simulink model "robotaz00"  (R2017a)
settings: Solver=VariableStepAuto  StartTime=0.0  StopTime=10.0  RelTol=1e-3
undefined symbols (not defined in the file or in its folder): Antebrazo, BASE, BrazoCOPIA, Codo, Hombrocopia, mesa, robotaz, RootGround, RootPart
libraries: mblibv1 x41
settings Model: Creator=ckarl  LastModifiedBy=ckarl
settings SimMechanicsCC: VisOnUpdateDiagram=on  VisDuringSimulation=on

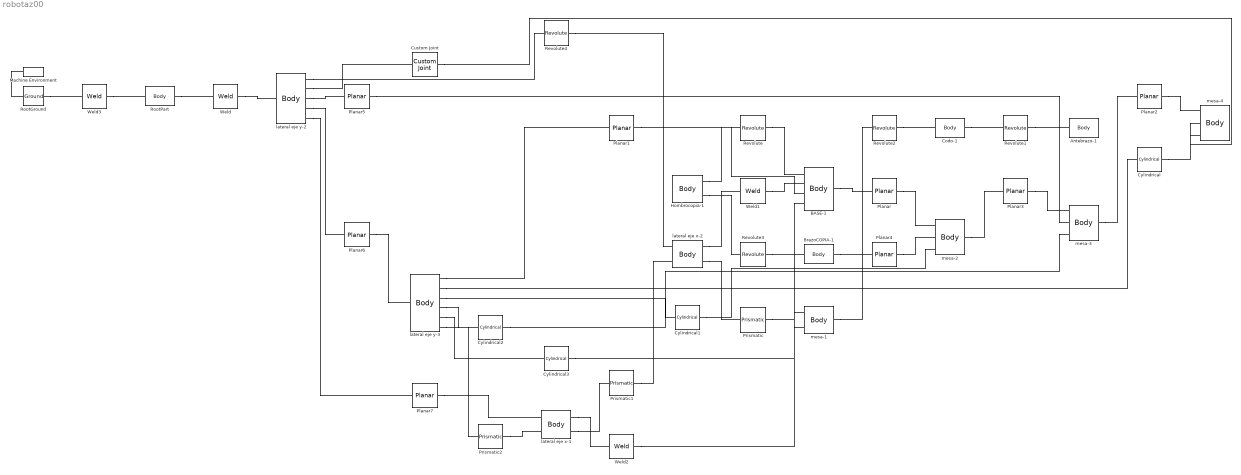
== system robotaz00 ==
  Antebrazo-1 : mblibv1/Bodies/Body  LConnTagsString=CS2  UpdateFromCAD=on  PMImportedID=Antebrazo-1  DialogClass=MechanicalBodyBlock  Mass=6.4203  MassUnits=kg  InertiaUnits=kg*m^2  Inertia=[0.103996,-2.98129e-06,0.00137963;-2.98129e-06,0.0987801,7.6206e-06;0.00137963,7.6206e-06,0.0190701]  Shape=Cylinder  ShapeDims=[1 1]  ShapeUnits=m  ShapeUse=false  Density=1  DensityUnits=kg/m^3  DensityUse=false  GraphicsMode=GFXFILE  GraphicsFileName=robotaz - Antebrazo-1.STL  BodyColorSelMode=COLORPALETTE  BodyColor=[0.792157;0.819608;0.933333]  AttachedToCS=CS1  CG=Right$CG$[-0.0536428 0.244253 1.19012]$WORLD$WORLD$m$[-0.573445 -0.772871 -0.271718;0.0436025 0.302406 -0.952181;0.818083 -0.557871 -0.139714]$3x3 Transform$rad$WORLD$false$Antebrazo-1::CG(AUTOGEN)  WorkingFrames=Right$CS1$[0.0431037 0.587411 1.24209]$WORLD$WORLD$m$[-0.573445 -0.772871 -0.271718;0.0436025 0.302406 -0.952181;0.818083 -0.557871 -0.139714]$3x3 Transform$rad$WORLD$false$Antebrazo-1::CS1(AUTOGEN)#Left$CS2$[0.000440757 0.437907 1.22016]$WORLD$WORLD$m$[1 0 0;0 1 0;0 0 1]$3x3 Transform$rad$WORLD$true$Antebrazo-1:-:Codo-1::Antebrazo-1(AUTOGEN)  CGPos=[-0.0536428 0.244253 1.19012]  CGRot=[-0.573445 -0.772871 -0.271718;0.0436025 0.302406 -0.952181;0.818083 -0.557871 -0.139714]  CS0Pos=[]  CS0Rot=[]  CS1Pos=[0.0431037 0.587411 1.24209]  CS1Rot=[-0.573445 -0.772871 -0.271718;0.0436025 0.302406 -0.952181;0.818083 -0.557871 -0.139714]  CS2Pos=[0.000440757 0.437907 1.22016]  CS2Rot=[1 0 0;0 1 0;0 0 1]  CS3Pos=[]  CS3Rot=[]  CS4Pos=[]  CS4Rot=[]  CS5Pos=[]  CS5Rot=[]  CS6Pos=[]  CS6Rot=[]  CS7Pos=[]  CS7Rot=[]  CS8Pos=[]  CS8Rot=[]  CS9Pos=[]  CS9Rot=[]  CS10Pos=[]  CS10Rot=[]  CS11Pos=[]  CS11Rot=[]  CS12Pos=[]  CS12Rot=[]  CS13Pos=[]  CS13Rot=[]  CS14Pos=[]  CS14Rot=[]  CS15Pos=[]  CS15Rot=[]  CS16Pos=[]  CS16Rot=[]  CS17Pos=[]  CS17Rot=[]  CS18Pos=[]  CS18Rot=[]  CS19Pos=[]  CS19Rot=[]  CS20Pos=[]  CS20Rot=[]
      settings: SourceProductName=Simscape Multibody  SourceProductBaseCode=MS
  BASE-1 : mblibv1/Bodies/Body  LConnTagsString=CS2|CS3|CS5|CS6  RConnTagsString=CS4  UpdateFromCAD=on  PMImportedID=BASE-1  DialogClass=MechanicalBodyBlock  Mass=23.2061  MassUnits=kg  InertiaUnits=kg*m^2  Inertia=[0.362789,0.0180466,-0.00054238;0.0180466,0.257111,-0.000428667;-0.00054238,-0.000428667,0.35504]  Shape=Cylinder  ShapeDims=[1 1]  ShapeUnits=m  ShapeUse=false  Density=1  DensityUnits=kg/m^3  DensityUse=false  GraphicsMode=GFXFILE  GraphicsFileName=robotaz - BASE-1.STL  BodyColorSelMode=COLORPALETTE  BodyColor=[1;0.54902;0]  AttachedToCS=CS1  CG=Right$CG$[0.148607 0.398211 0.794801]$WORLD$WORLD$m$[1 0 0;0 1 0;0 0 1]$3x3 Transform$rad$WORLD$false$BASE-1::CG(AUTOGEN)  WorkingFrames=Right$CS1$[0.140125 0.230213 0.795]$WORLD$WORLD$m$[1 0 0;0 1 0;0 0 1]$3x3 Transform$rad$WORLD$false$BASE-1::CS1(AUTOGEN)#Left$CS2$[0.140125 0.580213 0.795]$WORLD$WORLD$m$[1 0 0;0 1 0;0 0 1]$3x3 Transform$rad$WORLD$true$BASE-1:-:Hombrocopia-1::BASE-1(AUTOGEN)#Left$CS3$[-0.0148746 0.0738361 0.795]$WORLD$WORLD$m$[1 0 0;0 1 0;0 0 1]$3x3 Transform$rad$WORLD$true$BASE-1:-:lateral eje x-2::BASE-1(AUTOGEN)#Right$CS4$[0.140125 0.230213 0.795]$WORLD$WORLD$m$[1 0 0;0 1 0;0 0 1]$3x3 Transform$rad$WORLD$true$BASE-1:-:mesa-2::BASE-1(AUTOGEN)#Left$CS5$[0.310125 -0.0917867 0.945]$WORLD$WORLD$m$[1 0 0;0 1 0;0 0 1]$3x3 Transform$rad$WORLD$true$BASE-1:-:lateral eje y-3::BASE-1(AUTOGEN)#Left$CS6$[0.295125 0.0738361 0.795]$WORLD$WORLD$m$[1 0 0;0 1 0;0 0 1]$3x3 Transform$rad$WORLD$true$BASE-1:-:lateral eje x-1::BASE-1(AUTOGEN)  CGPos=[0.148607 0.398211 0.794801]  CGRot=[1 0 0;0 1 0;0 0 1]  CS0Pos=[]  CS0Rot=[]  CS1Pos=[0.140125 0.230213 0.795]  CS1Rot=[1 0 0;0 1 0;0 0 1]  CS2Pos=[0.140125 0.580213 0.795]  CS2Rot=[1 0 0;0 1 0;0 0 1]  CS3Pos=[-0.0148746 0.0738361 0.795]  CS3Rot=[1 0 0;0 1 0;0 0 1]  CS4Pos=[0.140125 0.230213 0.795]  CS4Rot=[1 0 0;0 1 0;0 0 1]  CS5Pos=[0.310125 -0.0917867 0.945]  CS5Rot=[1 0 0;0 1 0;0 0 1]  CS6Pos=[0.295125 0.0738361 0.795]  CS6Rot=[1 0 0;0 1 0;0 0 1]  CS7Pos=[]  CS7Rot=[]  CS8Pos=[]  CS8Rot=[]  CS9Pos=[]  CS9Rot=[]  CS10Pos=[]  CS10Rot=[]  CS11Pos=[]  CS11Rot=[]  CS12Pos=[]  CS12Rot=[]  CS13Pos=[]  CS13Rot=[]  CS14Pos=[]  CS14Rot=[]  CS15Pos=[]  CS15Rot=[]  CS16Pos=[]  CS16Rot=[]  CS17Pos=[]  CS17Rot=[]  CS18Pos=[]  CS18Rot=[]  CS19Pos=[]  CS19Rot=[]  CS20Pos=[]  CS20Rot=[]
      settings: SourceProductName=Simscape Multibody  SourceProductBaseCode=MS
  BrazoCOPIA-1 : mblibv1/Bodies/Body  LConnTagsString=CS3  RConnTagsString=CS2  UpdateFromCAD=on  PMImportedID=BrazoCOPIA-1  DialogClass=MechanicalBodyBlock  Mass=31.6067  MassUnits=kg  InertiaUnits=kg*m^2  Inertia=[3.43366,-7.27901e-06,-0.0175763;-7.27901e-06,3.34876,-4.89263e-05;-0.0175763,-4.89263e-05,0.211578]  Shape=Cylinder  ShapeDims=[1 1]  ShapeUnits=m  ShapeUse=false  Density=1  DensityUnits=kg/m^3  DensityUse=false  GraphicsMode=GFXFILE  GraphicsFileName=robotaz - BrazoCOPIA-1.STL  BodyColorSelMode=COLORPALETTE  BodyColor=[0.792157;0.819608;0.933333]  AttachedToCS=CS1  CG=Right$CG$[-0.109909 1.05734 1.38561]$WORLD$WORLD$m$[0.45728 -0.87962 -0.131012;0 -0.147317 0.989089;-0.889323 -0.45229 -0.067365]$3x3 Transform$rad$WORLD$false$BrazoCOPIA-1::CG(AUTOGEN)  WorkingFrames=Right$CS1$[-0.15801 1.37772 1.37482]$WORLD$WORLD$m$[0.45728 -0.87962 -0.131012;0 -0.147317 0.989089;-0.889323 -0.45229 -0.067365]$3x3 Transform$rad$WORLD$false$BrazoCOPIA-1::CS1(AUTOGEN)#Right$CS2$[-0.0120448 0.586448 1.34867]$WORLD$WORLD$m$[1 0 0;0 1 0;0 0 1]$3x3 Transform$rad$WORLD$true$BrazoCOPIA-1:-:Codo-1::BrazoCOPIA-1(AUTOGEN)#Left$CS3$[-0.116855 1.37772 1.29478]$WORLD$WORLD$m$[1 0 0;0 1 0;0 0 1]$3x3 Transform$rad$WORLD$true$BrazoCOPIA-1:-:Hombrocopia-1::BrazoCOPIA-1(AUTOGEN)  CGPos=[-0.109909 1.05734 1.38561]  CGRot=[0.45728 -0.87962 -0.131012;0 -0.147317 0.989089;-0.889323 -0.45229 -0.067365]  CS0Pos=[]  CS0Rot=[]  CS1Pos=[-0.15801 1.37772 1.37482]  CS1Rot=[0.45728 -0.87962 -0.131012;0 -0.147317 0.989089;-0.889323 -0.45229 -0.067365]  CS2Pos=[-0.0120448 0.586448 1.34867]  CS2Rot=[1 0 0;0 1 0;0 0 1]  CS3Pos=[-0.116855 1.37772 1.29478]  CS3Rot=[1 0 0;0 1 0;0 0 1]  CS4Pos=[]  CS4Rot=[]  CS5Pos=[]  CS5Rot=[]  CS6Pos=[]  CS6Rot=[]  CS7Pos=[]  CS7Rot=[]  CS8Pos=[]  CS8Rot=[]  CS9Pos=[]  CS9Rot=[]  CS10Pos=[]  CS10Rot=[]  CS11Pos=[]  CS11Rot=[]  CS12Pos=[]  CS12Rot=[]  CS13Pos=[]  CS13Rot=[]  CS14Pos=[]  CS14Rot=[]  CS15Pos=[]  CS15Rot=[]  CS16Pos=[]  CS16Rot=[]  CS17Pos=[]  CS17Rot=[]  CS18Pos=[]  CS18Rot=[]  CS19Pos=[]  CS19Rot=[]  CS20Pos=[]  CS20Rot=[]
      settings: SourceProductName=Simscape Multibody  SourceProductBaseCode=MS
  Codo-1 : mblibv1/Bodies/Body  LConnTagsString=CS3  RConnTagsString=CS2  UpdateFromCAD=on  PMImportedID=Codo-1  DialogClass=MechanicalBodyBlock  Mass=7.50271  MassUnits=kg  InertiaUnits=kg*m^2  Inertia=[0.0589129,-4.83716e-07,4.92094e-07;-4.83716e-07,0.0342772,-0.00366648;4.92094e-07,-0.00366648,0.0568936]  Shape=Cylinder  ShapeDims=[1 1]  ShapeUnits=m  ShapeUse=false  Density=1  DensityUnits=kg/m^3  DensityUse=false  GraphicsMode=GFXFILE  GraphicsFileName=robotaz - Codo-1.STL  BodyColorSelMode=COLORPALETTE  BodyColor=[0.792157;0.819608;0.933333]  AttachedToCS=CS1  CG=Right$CG$[0.0349873 0.583035 1.2548]$WORLD$WORLD$m$[0.846797 0.271718 -0.45728;-0.305534 0.952181 0;0.435413 0.139714 0.889323]$3x3 Transform$rad$WORLD$false$Codo-1::CG(AUTOGEN)  WorkingFrames=Right$CS1$[0.0428288 0.586448 1.24195]$WORLD$WORLD$m$[0.846797 0.271718 -0.45728;-0.305534 0.952181 0;0.435413 0.139714 0.889323]$3x3 Transform$rad$WORLD$false$Codo-1::CS1(AUTOGEN)#Right$CS2$[0.000440757 0.437907 1.22016]$WORLD$WORLD$m$[1 0 0;0 1 0;0 0 1]$3x3 Transform$rad$WORLD$true$Antebrazo-1:-:Codo-1::Codo-1(AUTOGEN)#Left$CS3$[-0.0120448 0.586448 1.34867]$WORLD$WORLD$m$[1 0 0;0 1 0;0 0 1]$3x3 Transform$rad$WORLD$true$BrazoCOPIA-1:-:Codo-1::Codo-1(AUTOGEN)  CGPos=[0.0349873 0.583035 1.2548]  CGRot=[0.846797 0.271718 -0.45728;-0.305534 0.952181 0;0.435413 0.139714 0.889323]  CS0Pos=[]  CS0Rot=[]  CS1Pos=[0.0428288 0.586448 1.24195]  CS1Rot=[0.846797 0.271718 -0.45728;-0.305534 0.952181 0;0.435413 0.139714 0.889323]  CS2Pos=[0.000440757 0.437907 1.22016]  CS2Rot=[1 0 0;0 1 0;0 0 1]  CS3Pos=[-0.0120448 0.586448 1.34867]  CS3Rot=[1 0 0;0 1 0;0 0 1]  CS4Pos=[]  CS4Rot=[]  CS5Pos=[]  CS5Rot=[]  CS6Pos=[]  CS6Rot=[]  CS7Pos=[]  CS7Rot=[]  CS8Pos=[]  CS8Rot=[]  CS9Pos=[]  CS9Rot=[]  CS10Pos=[]  CS10Rot=[]  CS11Pos=[]  CS11Rot=[]  CS12Pos=[]  CS12Rot=[]  CS13Pos=[]  CS13Rot=[]  CS14Pos=[]  CS14Rot=[]  CS15Pos=[]  CS15Rot=[]  CS16Pos=[]  CS16Rot=[]  CS17Pos=[]  CS17Rot=[]  CS18Pos=[]  CS18Rot=[]  CS19Pos=[]  CS19Rot=[]  CS20Pos=[]  CS20Rot=[]
      settings: SourceProductName=Simscape Multibody  SourceProductBaseCode=MS
  Custom Joint : mblibv1/Joints/Custom Joint  LConnTagsString=__newl0  RConnTagsString=__newr0  UpdateFromCAD=on  PMImportedID=lateral eje y-2:-:mesa-4  NumSAPorts=0  CutJoint=off  MarkAsCut=off  Primitives=prismatic  PrimitiveProps=P1$WORLD$[1,0,0]$prismatic#P2$WORLD$[0,1,0]$prismatic#P3$WORLD$[0,0,1]$prismatic#R1$WORLD$[0,1,0]$revolute  DialogClass=JointBlock  R1Axis=[0,1,0]  R2Axis=[]  R3Axis=[]  P1Axis=[1,0,0]  P2Axis=[0,1,0]  P3Axis=[0,0,1]  SAxis=[]
      settings: SourceProductName=Simscape Multibody  SourceProductBaseCode=MS
  Cylindrical : mblibv1/Joints/Cylindrical  LConnTagsString=__newl0  RConnTagsString=__newr0  UpdateFromCAD=on  PMImportedID=lateral eje y-3:-:mesa-4  NumSAPorts=0  CutJoint=off  MarkAsCut=off  Primitives=prismatic  PrimitiveProps=P1$WORLD$[1,0,0]$prismatic#R1$WORLD$[-1,0,0]$revolute  DialogClass=JointBlock  P1Axis=[1,0,0]  R1Axis=[-1,0,0]
      settings: SourceProductName=Simscape Multibody  SourceProductBaseCode=MS
  Cylindrical1 : mblibv1/Joints/Cylindrical  LConnTagsString=__newl0  RConnTagsString=__newr0  UpdateFromCAD=on  PMImportedID=lateral eje y-3:-:mesa-2  NumSAPorts=0  CutJoint=off  MarkAsCut=off  Primitives=prismatic  PrimitiveProps=P1$WORLD$[1,0,0]$prismatic#R1$WORLD$[-1,0,0]$revolute  DialogClass=JointBlock  P1Axis=[1,0,0]  R1Axis=[-1,0,0]
      settings: SourceProductName=Simscape Multibody  SourceProductBaseCode=MS
  Cylindrical2 : mblibv1/Joints/Cylindrical  LConnTagsString=__newl0  RConnTagsString=__newr0  UpdateFromCAD=on  PMImportedID=lateral eje y-3:-:mesa-3  NumSAPorts=0  CutJoint=off  MarkAsCut=off  Primitives=prismatic  PrimitiveProps=P1$WORLD$[1,0,0]$prismatic#R1$WORLD$[-1,0,0]$revolute  DialogClass=JointBlock  P1Axis=[1,0,0]  R1Axis=[-1,0,0]
      settings: SourceProductName=Simscape Multibody  SourceProductBaseCode=MS
  Cylindrical3 : mblibv1/Joints/Cylindrical  LConnTagsString=__newl0  RConnTagsString=__newr0  UpdateFromCAD=on  PMImportedID=lateral eje y-3:-:mesa-1  NumSAPorts=0  CutJoint=off  MarkAsCut=off  Primitives=prismatic  PrimitiveProps=P1$WORLD$[1,0,0]$prismatic#R1$WORLD$[-1,0,0]$revolute  DialogClass=JointBlock  P1Axis=[1,0,0]  R1Axis=[-1,0,0]
      settings: SourceProductName=Simscape Multibody  SourceProductBaseCode=MS
  Hombrocopia-1 : mblibv1/Bodies/Body  RConnTagsString=CS2|CS3  UpdateFromCAD=on  PMImportedID=Hombrocopia-1  DialogClass=MechanicalBodyBlock  Mass=67.0482  MassUnits=kg  InertiaUnits=kg*m^2  Inertia=[5.76162,2.80703,-1.87784e-05;2.80703,2.59803,1.32176e-05;-1.87784e-05,1.32176e-05,7.64234]  Shape=Cylinder  ShapeDims=[1 1]  ShapeUnits=m  ShapeUse=false  Density=1  DensityUnits=kg/m^3  DensityUse=false  GraphicsMode=GFXFILE  GraphicsFileName=robotaz - Hombrocopia-1.STL  BodyColorSelMode=COLORPALETTE  BodyColor=[0.792157;0.819608;0.933333]  AttachedToCS=CS1  CG=Right$CG$[0.0703324 1.06402 0.930737]$WORLD$WORLD$m$[0.45728 0 0.889323;0 1 0;-0.889323 0 0.45728]$3x3 Transform$rad$WORLD$false$Hombrocopia-1::CG(AUTOGEN)  WorkingFrames=Right$CS1$[0.140125 0.800213 0.795]$WORLD$WORLD$m$[0.45728 0 0.889323;0 1 0;-0.889323 0 0.45728]$3x3 Transform$rad$WORLD$false$Hombrocopia-1::CS1(AUTOGEN)#Right$CS2$[0.140125 0.580213 0.795]$WORLD$WORLD$m$[1 0 0;0 1 0;0 0 1]$3x3 Transform$rad$WORLD$true$BASE-1:-:Hombrocopia-1::Hombrocopia-1(AUTOGEN)#Right$CS3$[-0.116855 1.37772 1.29478]$WORLD$WORLD$m$[1 0 0;0 1 0;0 0 1]$3x3 Transform$rad$WORLD$true$BrazoCOPIA-1:-:Hombrocopia-1::Hombrocopia-1(AUTOGEN)  CGPos=[0.0703324 1.06402 0.930737]  CGRot=[0.45728 0 0.889323;0 1 0;-0.889323 0 0.45728]  CS0Pos=[]  CS0Rot=[]  CS1Pos=[0.140125 0.800213 0.795]  CS1Rot=[0.45728 0 0.889323;0 1 0;-0.889323 0 0.45728]  CS2Pos=[0.140125 0.580213 0.795]  CS2Rot=[1 0 0;0 1 0;0 0 1]  CS3Pos=[-0.116855 1.37772 1.29478]  CS3Rot=[1 0 0;0 1 0;0 0 1]  CS4Pos=[]  CS4Rot=[]  CS5Pos=[]  CS5Rot=[]  CS6Pos=[]  CS6Rot=[]  CS7Pos=[]  CS7Rot=[]  CS8Pos=[]  CS8Rot=[]  CS9Pos=[]  CS9Rot=[]  CS10Pos=[]  CS10Rot=[]  CS11Pos=[]  CS11Rot=[]  CS12Pos=[]  CS12Rot=[]  CS13Pos=[]  CS13Rot=[]  CS14Pos=[]  CS14Rot=[]  CS15Pos=[]  CS15Rot=[]  CS16Pos=[]  CS16Rot=[]  CS17Pos=[]  CS17Rot=[]  CS18Pos=[]  CS18Rot=[]  CS19Pos=[]  CS19Rot=[]  CS20Pos=[]  CS20Rot=[]
      settings: SourceProductName=Simscape Multibody  SourceProductBaseCode=MS
  Machine Environment : mblibv1/Bodies/Machine Environment  PortType=env  PhysicalDomain=Mechanical  DialogTemplateClass=MECH.MachineEnvironment  SyncWhenCopied=off  Gravity=[0 -9.81 0]  GravityUnits=m/s^2  GravityAsSignal=off  Dimensionality=Auto-detect  AnalysisType=Forward dynamics  LinearAssemblyTolerance=1e-3  LinearAssemblyToleranceUnits=m  AngularAssemblyTolerance=1e-3  AngularAssemblyToleranceUnits=rad  ConstraintSolverType=Stabilizing  ConstraintRelTolerance=1e-4  ConstraintAbsTolerance=1e-4  UseRobustSingularityHandling=off  RedundancyAnalysisToleranceType=Automatically select tolerance  RedundancyAnalysisTolerance=1e-14  StatePerturbationType=Fixed  PerturbationSize=1e-5  VisualizeMachine=on  BodyVisualizationType=Use model default body geometries  BodyColorSelMode=Use model default  DefaultBodyColor=[1 0 0]
      settings: SourceProductName=Simscape Multibody  SourceProductBaseCode=MS
  Planar : mblibv1/Joints/Planar  LConnTagsString=__newl0  RConnTagsString=__newr0  UpdateFromCAD=on  PMImportedID=BASE-1:-:mesa-2  NumSAPorts=0  CutJoint=off  MarkAsCut=off  Primitives=prismatic_prismatic  PrimitiveProps=P1$WORLD$[-1,0,0]$prismatic#P2$WORLD$[0,0,1]$prismatic#R1$WORLD$[0,-1,0]$revolute  DialogClass=JointBlock  P1Axis=[-1,0,0]  P2Axis=[0,0,1]  R1Axis=[0,-1,0]
      settings: SourceProductName=Simscape Multibody  SourceProductBaseCode=MS
  Planar1 : mblibv1/Joints/Planar  LConnTagsString=__newl0  RConnTagsString=__newr0  UpdateFromCAD=on  PMImportedID=BASE-1:-:lateral eje y-3  NumSAPorts=0  CutJoint=off  MarkAsCut=off  Primitives=prismatic_prismatic  PrimitiveProps=P1$WORLD$[-1,0,0]$prismatic#P2$WORLD$[0,-1,0]$prismatic#R1$WORLD$[0,0,-1]$revolute  DialogClass=JointBlock  P1Axis=[-1,0,0]  P2Axis=[0,-1,0]  R1Axis=[0,0,-1]
      settings: SourceProductName=Simscape Multibody  SourceProductBaseCode=MS
  Planar2 : mblibv1/Joints/Planar  LConnTagsString=__newl0  RConnTagsString=__newr0  UpdateFromCAD=on  PMImportedID=mesa-3:-:mesa-4  NumSAPorts=0  CutJoint=off  MarkAsCut=off  Primitives=prismatic_prismatic  PrimitiveProps=P1$WORLD$[0,-1,0]$prismatic#P2$WORLD$[0,0,1]$prismatic#R1$WORLD$[1,0,0]$revolute  DialogClass=JointBlock  P1Axis=[0,-1,0]  P2Axis=[0,0,1]  R1Axis=[1,0,0]
      settings: SourceProductName=Simscape Multibody  SourceProductBaseCode=MS
  Planar3 : mblibv1/Joints/Planar  LConnTagsString=__newl0  RConnTagsString=__newr0  UpdateFromCAD=on  PMImportedID=mesa-2:-:mesa-3  NumSAPorts=0  CutJoint=off  MarkAsCut=off  Primitives=prismatic_prismatic  PrimitiveProps=P1$WORLD$[0,-1,0]$prismatic#P2$WORLD$[0,0,1]$prismatic#R1$WORLD$[1,0,0]$revolute  DialogClass=JointBlock  P1Axis=[0,-1,0]  P2Axis=[0,0,1]  R1Axis=[1,0,0]
      settings: SourceProductName=Simscape Multibody  SourceProductBaseCode=MS
  Planar4 : mblibv1/Joints/Planar  LConnTagsString=__newl0  RConnTagsString=__newr0  UpdateFromCAD=on  PMImportedID=mesa-1:-:mesa-2  NumSAPorts=0  CutJoint=off  MarkAsCut=off  Primitives=prismatic_prismatic  PrimitiveProps=P1$WORLD$[0,-1,0]$prismatic#P2$WORLD$[0,0,1]$prismatic#R1$WORLD$[1,0,0]$revolute  DialogClass=JointBlock  P1Axis=[0,-1,0]  P2Axis=[0,0,1]  R1Axis=[1,0,0]
      settings: SourceProductName=Simscape Multibody  SourceProductBaseCode=MS
  Planar5 : mblibv1/Joints/Planar  LConnTagsString=__newl0  RConnTagsString=__newr0  UpdateFromCAD=on  PMImportedID=lateral eje y-2:-:mesa-3  NumSAPorts=0  CutJoint=off  MarkAsCut=off  Primitives=prismatic_prismatic  PrimitiveProps=P1$WORLD$[1,0,0]$prismatic#P2$WORLD$[0,0,1]$prismatic#R1$WORLD$[0,1,0]$revolute  DialogClass=JointBlock  P1Axis=[1,0,0]  P2Axis=[0,0,1]  R1Axis=[0,1,0]
      settings: SourceProductName=Simscape Multibody  SourceProductBaseCode=MS
  Planar6 : mblibv1/Joints/Planar  LConnTagsString=__newl0  RConnTagsString=__newr0  UpdateFromCAD=on  PMImportedID=lateral eje y-2:-:lateral eje y-3  NumSAPorts=0  CutJoint=off  MarkAsCut=off  Primitives=prismatic_prismatic  PrimitiveProps=P1$WORLD$[0,-1,0]$prismatic#P2$WORLD$[0,0,1]$prismatic#R1$WORLD$[-1,0,0]$revolute  DialogClass=JointBlock  P1Axis=[0,-1,0]  P2Axis=[0,0,1]  R1Axis=[-1,0,0]
      settings: SourceProductName=Simscape Multibody  SourceProductBaseCode=MS
  Planar7 : mblibv1/Joints/Planar  LConnTagsString=__newl0  RConnTagsString=__newr0  UpdateFromCAD=on  PMImportedID=lateral eje x-1:-:lateral eje y-2  NumSAPorts=0  CutJoint=off  MarkAsCut=off  Primitives=prismatic_prismatic  PrimitiveProps=P1$WORLD$[1,0,0]$prismatic#P2$WORLD$[0,0,1]$prismatic#R1$WORLD$[0,-1,0]$revolute  DialogClass=JointBlock  P1Axis=[1,0,0]  P2Axis=[0,0,1]  R1Axis=[0,-1,0]
      settings: SourceProductName=Simscape Multibody  SourceProductBaseCode=MS
  Prismatic : mblibv1/Joints/Prismatic  LConnTagsString=__newl0  RConnTagsString=__newr0  UpdateFromCAD=on  PMImportedID=lateral eje x-2:-:mesa-1  NumSAPorts=0  CutJoint=off  MarkAsCut=off  Primitives=prismatic  PrimitiveProps=P1$WORLD$[0,0,-1]$prismatic  DialogClass=JointBlock  P1Axis=[0,0,-1]
      settings: SourceProductName=Simscape Multibody  SourceProductBaseCode=MS
  Prismatic1 : mblibv1/Joints/Prismatic  LConnTagsString=__newl0  RConnTagsString=__newr0  UpdateFromCAD=on  PMImportedID=lateral eje x-1:-:lateral eje x-2  NumSAPorts=0  CutJoint=off  MarkAsCut=off  Primitives=prismatic  PrimitiveProps=P1$WORLD$[-1,0,0]$prismatic  DialogClass=JointBlock  P1Axis=[-1,0,0]
      settings: SourceProductName=Simscape Multibody  SourceProductBaseCode=MS
  Prismatic2 : mblibv1/Joints/Prismatic  LConnTagsString=__newl0  RConnTagsString=__newr0  UpdateFromCAD=on  PMImportedID=lateral eje x-1:-:lateral eje y-3  NumSAPorts=0  CutJoint=off  MarkAsCut=off  Primitives=prismatic  PrimitiveProps=P1$WORLD$[-1,0,0]$prismatic  DialogClass=JointBlock  P1Axis=[-1,0,0]
      settings: SourceProductName=Simscape Multibody  SourceProductBaseCode=MS
  Revolute : mblibv1/Joints/Revolute  LConnTagsString=__newl0  RConnTagsString=__newr0  UpdateFromCAD=on  PMImportedID=BASE-1:-:Hombrocopia-1  NumSAPorts=0  CutJoint=off  MarkAsCut=off  Primitives=prismatic  PrimitiveProps=R1$WORLD$[0,-1,0]$revolute  DialogClass=JointBlock  R1Axis=[0,-1,0]
      settings: SourceProductName=Simscape Multibody  SourceProductBaseCode=MS
  Revolute1 : mblibv1/Joints/Revolute  LConnTagsString=__newl0  RConnTagsString=__newr0  UpdateFromCAD=on  PMImportedID=Antebrazo-1:-:Codo-1  NumSAPorts=0  CutJoint=off  MarkAsCut=off  Primitives=prismatic  PrimitiveProps=R1$WORLD$[-0.271718,-0.952181,-0.139714]$revolute  DialogClass=JointBlock  R1Axis=[-0.271718,-0.952181,-0.139714]
      settings: SourceProductName=Simscape Multibody  SourceProductBaseCode=MS
  Revolute2 : mblibv1/Joints/Revolute  LConnTagsString=__newl0  RConnTagsString=__newr0  UpdateFromCAD=on  PMImportedID=BrazoCOPIA-1:-:Codo-1  NumSAPorts=0  CutJoint=off  MarkAsCut=off  Primitives=prismatic  PrimitiveProps=R1$WORLD$[0.45728,0,-0.889323]$revolute  DialogClass=JointBlock  R1Axis=[0.45728,0,-0.889323]
      settings: SourceProductName=Simscape Multibody  SourceProductBaseCode=MS
  Revolute3 : mblibv1/Joints/Revolute  LConnTagsString=__newl0  RConnTagsString=__newr0  UpdateFromCAD=on  PMImportedID=BrazoCOPIA-1:-:Hombrocopia-1  NumSAPorts=0  CutJoint=off  MarkAsCut=off  Primitives=prismatic  PrimitiveProps=R1$WORLD$[-0.45728,0,0.889323]$revolute  DialogClass=JointBlock  R1Axis=[-0.45728,0,0.889323]
      settings: SourceProductName=Simscape Multibody  SourceProductBaseCode=MS
  Revolute4 : mblibv1/Joints/Revolute  LConnTagsString=__newl0  RConnTagsString=__newr0  UpdateFromCAD=on  PMImportedID=lateral eje x-2:-:lateral eje y-2  NumSAPorts=0  CutJoint=off  MarkAsCut=off  Primitives=prismatic  PrimitiveProps=R1$WORLD$[0,0,1]$revolute  DialogClass=JointBlock  R1Axis=[0,0,1]
      settings: SourceProductName=Simscape Multibody  SourceProductBaseCode=MS
  RootGround : mblibv1/Bodies/Ground  UpdateFromCAD=on  PMImportedID=RootGround  LeftPortType=env  RightPortType=workingframe  PhysicalDomain=Mechanical  DialogClass=GroundBlock  CoordPosition=[0.0370155,0.859504,1.03604]  CoordPositionUnits=m  StateVectorMgrId=1  MachineId=[2 0]  ShowEnvPort=on  ParameterChecksum=[2454816870, 958179003, 3223168772, 3877319724]  TopologyChecksum=[1520872786, 2504460817, 446703565, 961653217]
      settings: SourceProductName=Simscape Multibody  SourceProductBaseCode=MS
  RootPart : mblibv1/Bodies/Body  LConnTagsString=CS3  RConnTagsString=CS2  UpdateFromCAD=on  PMImportedID=robotaz/RootPart  DialogClass=MechanicalBodyBlock  Mass=0  MassUnits=kg  InertiaUnits=kg*m^2  Inertia=[0,0,0;0,0,0;0,0,0]  Shape=Cylinder  ShapeDims=[1 1]  ShapeUnits=m  ShapeUse=false  Density=1  DensityUnits=kg/m^3  DensityUse=false  GraphicsMode=MACHINE_DEFAULT  BodyColorSelMode=MACHINE_DEFAULT  BodyColor=[1;0;0]  AttachedToCS=CS1  CG=Right$CG$[0.0370155 0.859504 1.03604]$WORLD$WORLD$m$[1 0 0;0 1 0;0 0 1]$3x3 Transform$rad$WORLD$false$robotaz/RootPart::CG(AUTOGEN)  WorkingFrames=Right$CS1$[0 0 0]$WORLD$WORLD$m$[1 0 0;0 1 0;0 0 1]$3x3 Transform$rad$WORLD$false$robotaz/RootPart::CS1(AUTOGEN)#Right$CS2$[0.129614 0.0667062 0.64]$WORLD$WORLD$m$[1 0 0;0 1 0;0 0 1]$3x3 Transform$rad$WORLD$true$lateral eje y-2:-:robotaz/RootPart::robotaz/RootPart(AUTOGEN)#Left$CS3$[0.0370155 0.859504 1.03604]$WORLD$WORLD$m$[1 0 0;0 1 0;0 0 1]$3x3 Transform$rad$WORLD$true$RootGround:-:robotaz/RootPart::robotaz/RootPart(AUTOGEN)  CGPos=[0.0370155 0.859504 1.03604]  CGRot=[1 0 0;0 1 0;0 0 1]  CS0Pos=[]  CS0Rot=[]  CS1Pos=[0 0 0]  CS1Rot=[1 0 0;0 1 0;0 0 1]  CS2Pos=[0.129614 0.0667062 0.64]  CS2Rot=[1 0 0;0 1 0;0 0 1]  CS3Pos=[0.0370155 0.859504 1.03604]  CS3Rot=[1 0 0;0 1 0;0 0 1]  CS4Pos=[]  CS4Rot=[]  CS5Pos=[]  CS5Rot=[]  CS6Pos=[]  CS6Rot=[]  CS7Pos=[]  CS7Rot=[]  CS8Pos=[]  CS8Rot=[]  CS9Pos=[]  CS9Rot=[]  CS10Pos=[]  CS10Rot=[]  CS11Pos=[]  CS11Rot=[]  CS12Pos=[]  CS12Rot=[]  CS13Pos=[]  CS13Rot=[]  CS14Pos=[]  CS14Rot=[]  CS15Pos=[]  CS15Rot=[]  CS16Pos=[]  CS16Rot=[]  CS17Pos=[]  CS17Rot=[]  CS18Pos=[]  CS18Rot=[]  CS19Pos=[]  CS19Rot=[]  CS20Pos=[]  CS20Rot=[]
      settings: SourceProductName=Simscape Multibody  SourceProductBaseCode=MS
  Weld : mblibv1/Joints/Weld  LConnTagsString=__newl0  RConnTagsString=__newr0  UpdateFromCAD=on  PMImportedID=lateral eje y-2:-:robotaz/RootPart  NumSAPorts=0  CutJoint=off  MarkAsCut=off  Primitives=weld  PrimitiveProps=W$WORLD$[0.57735,0.57735,0.57735]$weld  DialogClass=JointBlock  WAxis=[0.57735,0.57735,0.57735]
      settings: SourceProductName=Simscape Multibody  SourceProductBaseCode=MS
  Weld1 : mblibv1/Joints/Weld  LConnTagsString=__newl0  RConnTagsString=__newr0  UpdateFromCAD=on  PMImportedID=BASE-1:-:lateral eje x-2  NumSAPorts=0  CutJoint=off  MarkAsCut=off  Primitives=weld  PrimitiveProps=W$WORLD$[0.57735,0.57735,0.57735]$weld  DialogClass=JointBlock  WAxis=[0.57735,0.57735,0.57735]
      settings: SourceProductName=Simscape Multibody  SourceProductBaseCode=MS
  Weld2 : mblibv1/Joints/Weld  LConnTagsString=__newl0  RConnTagsString=__newr0  UpdateFromCAD=on  PMImportedID=BASE-1:-:lateral eje x-1  NumSAPorts=0  CutJoint=off  MarkAsCut=off  Primitives=weld  PrimitiveProps=W$WORLD$[0.57735,0.57735,0.57735]$weld  DialogClass=JointBlock  WAxis=[0.57735,0.57735,0.57735]
      settings: SourceProductName=Simscape Multibody  SourceProductBaseCode=MS
  Weld3 : mblibv1/Joints/Weld  LConnTagsString=__newl0  RConnTagsString=__newr0  UpdateFromCAD=on  PMImportedID=RootGround:-:robotaz/RootPart  NumSAPorts=0  CutJoint=off  MarkAsCut=off  Primitives=weld  PrimitiveProps=W$WORLD$[0.57735,0.57735,0.57735]$weld  DialogClass=JointBlock  WAxis=[0.57735,0.57735,0.57735]
      settings: SourceProductName=Simscape Multibody  SourceProductBaseCode=MS
  lateral eje x-1 : mblibv1/Bodies/Body  LConnTagsString=CS4|CS5  RConnTagsString=CS2|CS3  UpdateFromCAD=on  PMImportedID=lateral eje x-1  DialogClass=MechanicalBodyBlock  Mass=0.79546  MassUnits=kg  InertiaUnits=kg*m^2  Inertia=[0.00491999,0,0;0,0.00637652,0;0,0,0.0112832]  Shape=Cylinder  ShapeDims=[1 1]  ShapeUnits=m  ShapeUse=false  Density=1  DensityUnits=kg/m^3  DensityUse=false  GraphicsMode=GFXFILE  GraphicsFileName=robotaz - lateral eje x-1.STL  BodyColorSelMode=COLORPALETTE  BodyColor=[0.792157;0.819608;0.933333]  AttachedToCS=CS1  CG=Right$CG$[0.295125 0.0738361 0.795]$WORLD$WORLD$m$[0 0 1;0 1 0;-1 0 0]$3x3 Transform$rad$WORLD$false$lateral eje x-1::CG(AUTOGEN)  WorkingFrames=Right$CS1$[0.290125 -0.0917867 0.645]$WORLD$WORLD$m$[0 0 1;0 1 0;-1 0 0]$3x3 Transform$rad$WORLD$false$lateral eje x-1::CS1(AUTOGEN)#Right$CS2$[0.295125 0.0738361 0.795]$WORLD$WORLD$m$[1 0 0;0 1 0;0 0 1]$3x3 Transform$rad$WORLD$true$BASE-1:-:lateral eje x-1::lateral eje x-1(AUTOGEN)#Right$CS3$[0.300125 0.185213 0.925]$WORLD$WORLD$m$[1 0 0;0 1 0;0 0 1]$3x3 Transform$rad$WORLD$true$lateral eje x-1:-:lateral eje x-2::lateral eje x-1(AUTOGEN)#Left$CS4$[-0.0398746 -0.0917867 0.645]$WORLD$WORLD$m$[1 0 0;0 1 0;0 0 1]$3x3 Transform$rad$WORLD$true$lateral eje x-1:-:lateral eje y-2::lateral eje x-1(AUTOGEN)#Left$CS5$[0.300125 -0.0917867 0.945]$WORLD$WORLD$m$[1 0 0;0 1 0;0 0 1]$3x3 Transform$rad$WORLD$true$lateral eje x-1:-:lateral eje y-3::lateral eje x-1(AUTOGEN)  CGPos=[0.295125 0.0738361 0.795]  CGRot=[0 0 1;0 1 0;-1 0 0]  CS0Pos=[]  CS0Rot=[]  CS1Pos=[0.290125 -0.0917867 0.645]  CS1Rot=[0 0 1;0 1 0;-1 0 0]  CS2Pos=[0.295125 0.0738361 0.795]  CS2Rot=[1 0 0;0 1 0;0 0 1]  CS3Pos=[0.300125 0.185213 0.925]  CS3Rot=[1 0 0;0 1 0;0 0 1]  CS4Pos=[-0.0398746 -0.0917867 0.645]  CS4Rot=[1 0 0;0 1 0;0 0 1]  CS5Pos=[0.300125 -0.0917867 0.945]  CS5Rot=[1 0 0;0 1 0;0 0 1]  CS6Pos=[]  CS6Rot=[]  CS7Pos=[]  CS7Rot=[]  CS8Pos=[]  CS8Rot=[]  CS9Pos=[]  CS9Rot=[]  CS10Pos=[]  CS10Rot=[]  CS11Pos=[]  CS11Rot=[]  CS12Pos=[]  CS12Rot=[]  CS13Pos=[]  CS13Rot=[]  CS14Pos=[]  CS14Rot=[]  CS15Pos=[]  CS15Rot=[]  CS16Pos=[]  CS16Rot=[]  CS17Pos=[]  CS17Rot=[]  CS18Pos=[]  CS18Rot=[]  CS19Pos=[]  CS19Rot=[]  CS20Pos=[]  CS20Rot=[]
      settings: SourceProductName=Simscape Multibody  SourceProductBaseCode=MS
  lateral eje x-2 : mblibv1/Bodies/Body  LConnTagsString=CS4|CS5  RConnTagsString=CS2|CS3  UpdateFromCAD=on  PMImportedID=lateral eje x-2  DialogClass=MechanicalBodyBlock  Mass=0.79546  MassUnits=kg  InertiaUnits=kg*m^2  Inertia=[0.00491999,0,0;0,0.00637652,0;0,0,0.0112832]  Shape=Cylinder  ShapeDims=[1 1]  ShapeUnits=m  ShapeUse=false  Density=1  DensityUnits=kg/m^3  DensityUse=false  GraphicsMode=GFXFILE  GraphicsFileName=robotaz - lateral eje x-2.STL  BodyColorSelMode=COLORPALETTE  BodyColor=[0.792157;0.819608;0.933333]  AttachedToCS=CS1  CG=Right$CG$[-0.0148746 0.0738361 0.795]$WORLD$WORLD$m$[0 0 -1;0 1 0;1 0 0]$3x3 Transform$rad$WORLD$false$lateral eje x-2::CG(AUTOGEN)  WorkingFrames=Right$CS1$[-0.00987456 -0.0917867 0.945]$WORLD$WORLD$m$[0 0 -1;0 1 0;1 0 0]$3x3 Transform$rad$WORLD$false$lateral eje x-2::CS1(AUTOGEN)#Right$CS2$[-0.0148746 0.0738361 0.795]$WORLD$WORLD$m$[1 0 0;0 1 0;0 0 1]$3x3 Transform$rad$WORLD$true$BASE-1:-:lateral eje x-2::lateral eje x-2(AUTOGEN)#Right$CS3$[-0.0198746 0.208213 0.945]$WORLD$WORLD$m$[1 0 0;0 1 0;0 0 1]$3x3 Transform$rad$WORLD$true$lateral eje x-2:-:mesa-1::lateral eje x-2(AUTOGEN)#Left$CS4$[-0.00987456 0.208213 0.645]$WORLD$WORLD$m$[1 0 0;0 1 0;0 0 1]$3x3 Transform$rad$WORLD$true$lateral eje x-2:-:lateral eje y-2::lateral eje x-2(AUTOGEN)#Left$CS5$[-0.0198746 0.185213 0.925]$WORLD$WORLD$m$[1 0 0;0 1 0;0 0 1]$3x3 Transform$rad$WORLD$true$lateral eje x-1:-:lateral eje x-2::lateral eje x-2(AUTOGEN)  CGPos=[-0.0148746 0.0738361 0.795]  CGRot=[0 0 -1;0 1 0;1 0 0]  CS0Pos=[]  CS0Rot=[]  CS1Pos=[-0.00987456 -0.0917867 0.945]  CS1Rot=[0 0 -1;0 1 0;1 0 0]  CS2Pos=[-0.0148746 0.0738361 0.795]  CS2Rot=[1 0 0;0 1 0;0 0 1]  CS3Pos=[-0.0198746 0.208213 0.945]  CS3Rot=[1 0 0;0 1 0;0 0 1]  CS4Pos=[-0.00987456 0.208213 0.645]  CS4Rot=[1 0 0;0 1 0;0 0 1]  CS5Pos=[-0.0198746 0.185213 0.925]  CS5Rot=[1 0 0;0 1 0;0 0 1]  CS6Pos=[]  CS6Rot=[]  CS7Pos=[]  CS7Rot=[]  CS8Pos=[]  CS8Rot=[]  CS9Pos=[]  CS9Rot=[]  CS10Pos=[]  CS10Rot=[]  CS11Pos=[]  CS11Rot=[]  CS12Pos=[]  CS12Rot=[]  CS13Pos=[]  CS13Rot=[]  CS14Pos=[]  CS14Rot=[]  CS15Pos=[]  CS15Rot=[]  CS16Pos=[]  CS16Rot=[]  CS17Pos=[]  CS17Rot=[]  CS18Pos=[]  CS18Rot=[]  CS19Pos=[]  CS19Rot=[]  CS20Pos=[]  CS20Rot=[]
      settings: SourceProductName=Simscape Multibody  SourceProductBaseCode=MS
  lateral eje y-2 : mblibv1/Bodies/Body  LConnTagsString=CS2  RConnTagsString=CS3|CS4|CS5|CS6|CS7  UpdateFromCAD=on  PMImportedID=lateral eje y-2  DialogClass=MechanicalBodyBlock  Mass=0.963525  MassUnits=kg  InertiaUnits=kg*m^2  Inertia=[0.0063819,-0.000492021,0;-0.000492021,0.00982296,0;0,0,0.0161888]  Shape=Cylinder  ShapeDims=[1 1]  ShapeUnits=m  ShapeUse=false  Density=1  DensityUnits=kg/m^3  DensityUse=false  GraphicsMode=GFXFILE  GraphicsFileName=robotaz - lateral eje y-2.STL  BodyColorSelMode=COLORPALETTE  BodyColor=[0.792157;0.819608;0.933333]  AttachedToCS=CS1  CG=Right$CG$[0.129614 0.0667062 0.64]$WORLD$WORLD$m$[1 0 0;0 1 0;0 0 1]$3x3 Transform$rad$WORLD$false$lateral eje y-2::CG(AUTOGEN)  WorkingFrames=Right$CS1$[0.310125 -0.0917867 0.635]$WORLD$WORLD$m$[1 0 0;0 1 0;0 0 1]$3x3 Transform$rad$WORLD$false$lateral eje y-2::CS1(AUTOGEN)#Left$CS2$[0.129614 0.0667062 0.64]$WORLD$WORLD$m$[1 0 0;0 1 0;0 0 1]$3x3 Transform$rad$WORLD$true$lateral eje y-2:-:robotaz/RootPart::lateral eje y-2(AUTOGEN)#Right$CS3$[-0.00987456 0.208213 0.645]$WORLD$WORLD$m$[1 0 0;0 1 0;0 0 1]$3x3 Transform$rad$WORLD$true$lateral eje x-2:-:lateral eje y-2::lateral eje y-2(AUTOGEN)#Right$CS4$[-0.0398746 0.208213 0.645]$WORLD$WORLD$m$[1 0 0;0 1 0;0 0 1]$3x3 Transform$rad$WORLD$true$lateral eje y-2:-:mesa-4::lateral eje y-2(AUTOGEN)#Right$CS5$[-0.0398746 0.208213 0.645]$WORLD$WORLD$m$[1 0 0;0 1 0;0 0 1]$3x3 Transform$rad$WORLD$true$lateral eje y-2:-:mesa-3::lateral eje y-2(AUTOGEN)#Right$CS6$[-0.0398746 -0.0917867 0.645]$WORLD$WORLD$m$[1 0 0;0 1 0;0 0 1]$3x3 Transform$rad$WORLD$true$lateral eje y-2:-:lateral eje y-3::lateral eje y-2(AUTOGEN)#Right$CS7$[-0.0398746 -0.0917867 0.645]$WORLD$WORLD$m$[1 0 0;0 1 0;0 0 1]$3x3 Transform$rad$WORLD$true$lateral eje x-1:-:lateral eje y-2::lateral eje y-2(AUTOGEN)  CGPos=[0.129614 0.0667062 0.64]  CGRot=[1 0 0;0 1 0;0 0 1]  CS0Pos=[]  CS0Rot=[]  CS1Pos=[0.310125 -0.0917867 0.635]  CS1Rot=[1 0 0;0 1 0;0 0 1]  CS2Pos=[0.129614 0.0667062 0.64]  CS2Rot=[1 0 0;0 1 0;0 0 1]  CS3Pos=[-0.00987456 0.208213 0.645]  CS3Rot=[1 0 0;0 1 0;0 0 1]  CS4Pos=[-0.0398746 0.208213 0.645]  CS4Rot=[1 0 0;0 1 0;0 0 1]  CS5Pos=[-0.0398746 0.208213 0.645]  CS5Rot=[1 0 0;0 1 0;0 0 1]  CS6Pos=[-0.0398746 -0.0917867 0.645]  CS6Rot=[1 0 0;0 1 0;0 0 1]  CS7Pos=[-0.0398746 -0.0917867 0.645]  CS7Rot=[1 0 0;0 1 0;0 0 1]  CS8Pos=[]  CS8Rot=[]  CS9Pos=[]  CS9Rot=[]  CS10Pos=[]  CS10Rot=[]  CS11Pos=[]  CS11Rot=[]  CS12Pos=[]  CS12Rot=[]  CS13Pos=[]  CS13Rot=[]  CS14Pos=[]  CS14Rot=[]  CS15Pos=[]  CS15Rot=[]  CS16Pos=[]  CS16Rot=[]  CS17Pos=[]  CS17Rot=[]  CS18Pos=[]  CS18Rot=[]  CS19Pos=[]  CS19Rot=[]  CS20Pos=[]  CS20Rot=[]
      settings: SourceProductName=Simscape Multibody  SourceProductBaseCode=MS
  lateral eje y-3 : mblibv1/Bodies/Body  LConnTagsString=CS7  RConnTagsString=CS2|CS3|CS4|CS5|CS6|CS8  UpdateFromCAD=on  PMImportedID=lateral eje y-3  DialogClass=MechanicalBodyBlock  Mass=0.963525  MassUnits=kg  InertiaUnits=kg*m^2  Inertia=[0.0063819,-0.000492021,0;-0.000492021,0.00982296,0;0,0,0.0161888]  Shape=Cylinder  ShapeDims=[1 1]  ShapeUnits=m  ShapeUse=false  Density=1  DensityUnits=kg/m^3  DensityUse=false  GraphicsMode=GFXFILE  GraphicsFileName=robotaz - lateral eje y-3.STL  BodyColorSelMode=COLORPALETTE  BodyColor=[0.792157;0.819608;0.933333]  AttachedToCS=CS1  CG=Right$CG$[0.129614 0.0667062 0.95]$WORLD$WORLD$m$[1 0 0;0 1 0;0 0 1]$3x3 Transform$rad$WORLD$false$lateral eje y-3::CG(AUTOGEN)  WorkingFrames=Right$CS1$[0.310125 -0.0917867 0.945]$WORLD$WORLD$m$[1 0 0;0 1 0;0 0 1]$3x3 Transform$rad$WORLD$false$lateral eje y-3::CS1(AUTOGEN)#Right$CS2$[0.310125 -0.0917867 0.945]$WORLD$WORLD$m$[1 0 0;0 1 0;0 0 1]$3x3 Transform$rad$WORLD$true$BASE-1:-:lateral eje y-3::lateral eje y-3(AUTOGEN)#Right$CS3$[0.280125 0.208213 0.945]$WORLD$WORLD$m$[1 0 0;0 1 0;0 0 1]$3x3 Transform$rad$WORLD$true$lateral eje y-3:-:mesa-4::lateral eje y-3(AUTOGEN)#Right$CS4$[0.280125 0.208213 0.945]$WORLD$WORLD$m$[1 0 0;0 1 0;0 0 1]$3x3 Transform$rad$WORLD$true$lateral eje y-3:-:mesa-2::lateral eje y-3(AUTOGEN)#Right$CS5$[0.280125 0.208213 0.945]$WORLD$WORLD$m$[1 0 0;0 1 0;0 0 1]$3x3 Transform$rad$WORLD$true$lateral eje y-3:-:mesa-3::lateral eje y-3(AUTOGEN)#Right$CS6$[0.280125 0.208213 0.945]$WORLD$WORLD$m$[1 0 0;0 1 0;0 0 1]$3x3 Transform$rad$WORLD$true$lateral eje y-3:-:mesa-1::lateral eje y-3(AUTOGEN)#Left$CS7$[-0.0398746 -0.0917867 0.645]$WORLD$WORLD$m$[1 0 0;0 1 0;0 0 1]$3x3 Transform$rad$WORLD$true$lateral eje y-2:-:lateral eje y-3::lateral eje y-3(AUTOGEN)#Right$CS8$[0.310125 -0.0917867 0.945]$WORLD$WORLD$m$[1 0 0;0 1 0;0 0 1]$3x3 Transform$rad$WORLD$true$lateral eje x-1:-:lateral eje y-3::lateral eje y-3(AUTOGEN)  CGPos=[0.129614 0.0667062 0.95]  CGRot=[1 0 0;0 1 0;0 0 1]  CS0Pos=[]  CS0Rot=[]  CS1Pos=[0.310125 -0.0917867 0.945]  CS1Rot=[1 0 0;0 1 0;0 0 1]  CS2Pos=[0.310125 -0.0917867 0.945]  CS2Rot=[1 0 0;0 1 0;0 0 1]  CS3Pos=[0.280125 0.208213 0.945]  CS3Rot=[1 0 0;0 1 0;0 0 1]  CS4Pos=[0.280125 0.208213 0.945]  CS4Rot=[1 0 0;0 1 0;0 0 1]  CS5Pos=[0.280125 0.208213 0.945]  CS5Rot=[1 0 0;0 1 0;0 0 1]  CS6Pos=[0.280125 0.208213 0.945]  CS6Rot=[1 0 0;0 1 0;0 0 1]  CS7Pos=[-0.0398746 -0.0917867 0.645]  CS7Rot=[1 0 0;0 1 0;0 0 1]  CS8Pos=[0.310125 -0.0917867 0.945]  CS8Rot=[1 0 0;0 1 0;0 0 1]  CS9Pos=[]  CS9Rot=[]  CS10Pos=[]  CS10Rot=[]  CS11Pos=[]  CS11Rot=[]  CS12Pos=[]  CS12Rot=[]  CS13Pos=[]  CS13Rot=[]  CS14Pos=[]  CS14Rot=[]  CS15Pos=[]  CS15Rot=[]  CS16Pos=[]  CS16Rot=[]  CS17Pos=[]  CS17Rot=[]  CS18Pos=[]  CS18Rot=[]  CS19Pos=[]  CS19Rot=[]  CS20Pos=[]  CS20Rot=[]
      settings: SourceProductName=Simscape Multibody  SourceProductBaseCode=MS
  mesa-1 : mblibv1/Bodies/Body  LConnTagsString=CS2|CS4  RConnTagsString=CS3  UpdateFromCAD=on  PMImportedID=mesa-1  DialogClass=MechanicalBodyBlock  Mass=0.178824  MassUnits=kg  InertiaUnits=kg*m^2  Inertia=[0.00135097,6.92632e-10,0;6.92632e-10,0.00144796,0;0,0,0.000116564]  Shape=Cylinder  ShapeDims=[1 1]  ShapeUnits=m  ShapeUse=false  Density=1  DensityUnits=kg/m^3  DensityUse=false  GraphicsMode=GFXFILE  GraphicsFileName=robotaz - mesa-1.STL  BodyColorSelMode=COLORPALETTE  BodyColor=[0.792157;0.819608;0.933333]  AttachedToCS=CS1  CG=Right$CG$[0.0191254 0.218601 0.795]$WORLD$WORLD$m$[1 0 0;0 1 0;0 0 1]$3x3 Transform$rad$WORLD$false$mesa-1::CG(AUTOGEN)  WorkingFrames=Right$CS1$[0.019168 0.219171 0.595]$WORLD$WORLD$m$[1 0 0;0 1 0;0 0 1]$3x3 Transform$rad$WORLD$false$mesa-1::CS1(AUTOGEN)#Left$CS2$[-0.0198746 0.208213 0.945]$WORLD$WORLD$m$[1 0 0;0 1 0;0 0 1]$3x3 Transform$rad$WORLD$true$lateral eje x-2:-:mesa-1::mesa-1(AUTOGEN)#Right$CS3$[0.0601254 0.210213 0.945]$WORLD$WORLD$m$[1 0 0;0 1 0;0 0 1]$3x3 Transform$rad$WORLD$true$mesa-1:-:mesa-2::mesa-1(AUTOGEN)#Left$CS4$[0.280125 0.208213 0.945]$WORLD$WORLD$m$[1 0 0;0 1 0;0 0 1]$3x3 Transform$rad$WORLD$true$lateral eje y-3:-:mesa-1::mesa-1(AUTOGEN)  CGPos=[0.0191254 0.218601 0.795]  CGRot=[1 0 0;0 1 0;0 0 1]  CS0Pos=[]  CS0Rot=[]  CS1Pos=[0.019168 0.219171 0.595]  CS1Rot=[1 0 0;0 1 0;0 0 1]  CS2Pos=[-0.0198746 0.208213 0.945]  CS2Rot=[1 0 0;0 1 0;0 0 1]  CS3Pos=[0.0601254 0.210213 0.945]  CS3Rot=[1 0 0;0 1 0;0 0 1]  CS4Pos=[0.280125 0.208213 0.945]  CS4Rot=[1 0 0;0 1 0;0 0 1]  CS5Pos=[]  CS5Rot=[]  CS6Pos=[]  CS6Rot=[]  CS7Pos=[]  CS7Rot=[]  CS8Pos=[]  CS8Rot=[]  CS9Pos=[]  CS9Rot=[]  CS10Pos=[]  CS10Rot=[]  CS11Pos=[]  CS11Rot=[]  CS12Pos=[]  CS12Rot=[]  CS13Pos=[]  CS13Rot=[]  CS14Pos=[]  CS14Rot=[]  CS15Pos=[]  CS15Rot=[]  CS16Pos=[]  CS16Rot=[]  CS17Pos=[]  CS17Rot=[]  CS18Pos=[]  CS18Rot=[]  CS19Pos=[]  CS19Rot=[]  CS20Pos=[]  CS20Rot=[]
      settings: SourceProductName=Simscape Multibody  SourceProductBaseCode=MS
  mesa-2 : mblibv1/Bodies/Body  LConnTagsString=CS2|CS4|CS5  RConnTagsString=CS3  UpdateFromCAD=on  PMImportedID=mesa-2  DialogClass=MechanicalBodyBlock  Mass=0.178824  MassUnits=kg  InertiaUnits=kg*m^2  Inertia=[0.00135097,6.92632e-10,0;6.92632e-10,0.00144796,0;0,0,0.000116564]  Shape=Cylinder  ShapeDims=[1 1]  ShapeUnits=m  ShapeUse=false  Density=1  DensityUnits=kg/m^3  DensityUse=false  GraphicsMode=GFXFILE  GraphicsFileName=robotaz - mesa-2.STL  BodyColorSelMode=COLORPALETTE  BodyColor=[0.792157;0.819608;0.933333]  AttachedToCS=CS1  CG=Right$CG$[0.101125 0.218601 0.795]$WORLD$WORLD$m$[1 0 0;0 1 0;0 0 1]$3x3 Transform$rad$WORLD$false$mesa-2::CG(AUTOGEN)  WorkingFrames=Right$CS1$[0.101168 0.219171 0.595]$WORLD$WORLD$m$[1 0 0;0 1 0;0 0 1]$3x3 Transform$rad$WORLD$false$mesa-2::CS1(AUTOGEN)#Left$CS2$[0.140125 0.230213 0.795]$WORLD$WORLD$m$[1 0 0;0 1 0;0 0 1]$3x3 Transform$rad$WORLD$true$BASE-1:-:mesa-2::mesa-2(AUTOGEN)#Right$CS3$[0.142125 0.210213 0.945]$WORLD$WORLD$m$[1 0 0;0 1 0;0 0 1]$3x3 Transform$rad$WORLD$true$mesa-2:-:mesa-3::mesa-2(AUTOGEN)#Left$CS4$[0.0601254 0.210213 0.945]$WORLD$WORLD$m$[1 0 0;0 1 0;0 0 1]$3x3 Transform$rad$WORLD$true$mesa-1:-:mesa-2::mesa-2(AUTOGEN)#Left$CS5$[0.280125 0.208213 0.945]$WORLD$WORLD$m$[1 0 0;0 1 0;0 0 1]$3x3 Transform$rad$WORLD$true$lateral eje y-3:-:mesa-2::mesa-2(AUTOGEN)  CGPos=[0.101125 0.218601 0.795]  CGRot=[1 0 0;0 1 0;0 0 1]  CS0Pos=[]  CS0Rot=[]  CS1Pos=[0.101168 0.219171 0.595]  CS1Rot=[1 0 0;0 1 0;0 0 1]  CS2Pos=[0.140125 0.230213 0.795]  CS2Rot=[1 0 0;0 1 0;0 0 1]  CS3Pos=[0.142125 0.210213 0.945]  CS3Rot=[1 0 0;0 1 0;0 0 1]  CS4Pos=[0.0601254 0.210213 0.945]  CS4Rot=[1 0 0;0 1 0;0 0 1]  CS5Pos=[0.280125 0.208213 0.945]  CS5Rot=[1 0 0;0 1 0;0 0 1]  CS6Pos=[]  CS6Rot=[]  CS7Pos=[]  CS7Rot=[]  CS8Pos=[]  CS8Rot=[]  CS9Pos=[]  CS9Rot=[]  CS10Pos=[]  CS10Rot=[]  CS11Pos=[]  CS11Rot=[]  CS12Pos=[]  CS12Rot=[]  CS13Pos=[]  CS13Rot=[]  CS14Pos=[]  CS14Rot=[]  CS15Pos=[]  CS15Rot=[]  CS16Pos=[]  CS16Rot=[]  CS17Pos=[]  CS17Rot=[]  CS18Pos=[]  CS18Rot=[]  CS19Pos=[]  CS19Rot=[]  CS20Pos=[]  CS20Rot=[]
      settings: SourceProductName=Simscape Multibody  SourceProductBaseCode=MS
  mesa-3 : mblibv1/Bodies/Body  LConnTagsString=CS3|CS4|CS5  RConnTagsString=CS2  UpdateFromCAD=on  PMImportedID=mesa-3  DialogClass=MechanicalBodyBlock  Mass=0.178824  MassUnits=kg  InertiaUnits=kg*m^2  Inertia=[0.00135097,6.92632e-10,0;6.92632e-10,0.00144796,0;0,0,0.000116564]  Shape=Cylinder  ShapeDims=[1 1]  ShapeUnits=m  ShapeUse=false  Density=1  DensityUnits=kg/m^3  DensityUse=false  GraphicsMode=GFXFILE  GraphicsFileName=robotaz - mesa-3.STL  BodyColorSelMode=COLORPALETTE  BodyColor=[0.792157;0.819608;0.933333]  AttachedToCS=CS1  CG=Right$CG$[0.183125 0.218601 0.795]$WORLD$WORLD$m$[1 0 0;0 1 0;0 0 1]$3x3 Transform$rad$WORLD$false$mesa-3::CG(AUTOGEN)  WorkingFrames=Right$CS1$[0.183168 0.219171 0.595]$WORLD$WORLD$m$[1 0 0;0 1 0;0 0 1]$3x3 Transform$rad$WORLD$false$mesa-3::CS1(AUTOGEN)#Right$CS2$[0.224125 0.210213 0.945]$WORLD$WORLD$m$[1 0 0;0 1 0;0 0 1]$3x3 Transform$rad$WORLD$true$mesa-3:-:mesa-4::mesa-3(AUTOGEN)#Left$CS3$[0.142125 0.210213 0.945]$WORLD$WORLD$m$[1 0 0;0 1 0;0 0 1]$3x3 Transform$rad$WORLD$true$mesa-2:-:mesa-3::mesa-3(AUTOGEN)#Left$CS4$[-0.0398746 0.208213 0.645]$WORLD$WORLD$m$[1 0 0;0 1 0;0 0 1]$3x3 Transform$rad$WORLD$true$lateral eje y-2:-:mesa-3::mesa-3(AUTOGEN)#Left$CS5$[0.280125 0.208213 0.945]$WORLD$WORLD$m$[1 0 0;0 1 0;0 0 1]$3x3 Transform$rad$WORLD$true$lateral eje y-3:-:mesa-3::mesa-3(AUTOGEN)  CGPos=[0.183125 0.218601 0.795]  CGRot=[1 0 0;0 1 0;0 0 1]  CS0Pos=[]  CS0Rot=[]  CS1Pos=[0.183168 0.219171 0.595]  CS1Rot=[1 0 0;0 1 0;0 0 1]  CS2Pos=[0.224125 0.210213 0.945]  CS2Rot=[1 0 0;0 1 0;0 0 1]  CS3Pos=[0.142125 0.210213 0.945]  CS3Rot=[1 0 0;0 1 0;0 0 1]  CS4Pos=[-0.0398746 0.208213 0.645]  CS4Rot=[1 0 0;0 1 0;0 0 1]  CS5Pos=[0.280125 0.208213 0.945]  CS5Rot=[1 0 0;0 1 0;0 0 1]  CS6Pos=[]  CS6Rot=[]  CS7Pos=[]  CS7Rot=[]  CS8Pos=[]  CS8Rot=[]  CS9Pos=[]  CS9Rot=[]  CS10Pos=[]  CS10Rot=[]  CS11Pos=[]  CS11Rot=[]  CS12Pos=[]  CS12Rot=[]  CS13Pos=[]  CS13Rot=[]  CS14Pos=[]  CS14Rot=[]  CS15Pos=[]  CS15Rot=[]  CS16Pos=[]  CS16Rot=[]  CS17Pos=[]  CS17Rot=[]  CS18Pos=[]  CS18Rot=[]  CS19Pos=[]  CS19Rot=[]  CS20Pos=[]  CS20Rot=[]
      settings: SourceProductName=Simscape Multibody  SourceProductBaseCode=MS
  mesa-4 : mblibv1/Bodies/Body  LConnTagsString=CS2|CS3|CS4  UpdateFromCAD=on  PMImportedID=mesa-4  DialogClass=MechanicalBodyBlock  Mass=0.178824  MassUnits=kg  InertiaUnits=kg*m^2  Inertia=[0.00135097,6.92632e-10,0;6.92632e-10,0.00144796,0;0,0,0.000116564]  Shape=Cylinder  ShapeDims=[1 1]  ShapeUnits=m  ShapeUse=false  Density=1  DensityUnits=kg/m^3  DensityUse=false  GraphicsMode=GFXFILE  GraphicsFileName=robotaz - mesa-4.STL  BodyColorSelMode=COLORPALETTE  BodyColor=[0.792157;0.819608;0.933333]  AttachedToCS=CS1  CG=Right$CG$[0.265125 0.217601 0.795]$WORLD$WORLD$m$[1 0 0;0 1 0;0 0 1]$3x3 Transform$rad$WORLD$false$mesa-4::CG(AUTOGEN)  WorkingFrames=Right$CS1$[0.265168 0.218171 0.595]$WORLD$WORLD$m$[1 0 0;0 1 0;0 0 1]$3x3 Transform$rad$WORLD$false$mesa-4::CS1(AUTOGEN)#Left$CS2$[0.224125 0.210213 0.945]$WORLD$WORLD$m$[1 0 0;0 1 0;0 0 1]$3x3 Transform$rad$WORLD$true$mesa-3:-:mesa-4::mesa-4(AUTOGEN)#Left$CS3$[-0.0398746 0.208213 0.645]$WORLD$WORLD$m$[1 0 0;0 1 0;0 0 1]$3x3 Transform$rad$WORLD$true$lateral eje y-2:-:mesa-4::mesa-4(AUTOGEN)#Left$CS4$[0.280125 0.208213 0.945]$WORLD$WORLD$m$[1 0 0;0 1 0;0 0 1]$3x3 Transform$rad$WORLD$true$lateral eje y-3:-:mesa-4::mesa-4(AUTOGEN)  CGPos=[0.265125 0.217601 0.795]  CGRot=[1 0 0;0 1 0;0 0 1]  CS0Pos=[]  CS0Rot=[]  CS1Pos=[0.265168 0.218171 0.595]  CS1Rot=[1 0 0;0 1 0;0 0 1]  CS2Pos=[0.224125 0.210213 0.945]  CS2Rot=[1 0 0;0 1 0;0 0 1]  CS3Pos=[-0.0398746 0.208213 0.645]  CS3Rot=[1 0 0;0 1 0;0 0 1]  CS4Pos=[0.280125 0.208213 0.945]  CS4Rot=[1 0 0;0 1 0;0 0 1]  CS5Pos=[]  CS5Rot=[]  CS6Pos=[]  CS6Rot=[]  CS7Pos=[]  CS7Rot=[]  CS8Pos=[]  CS8Rot=[]  CS9Pos=[]  CS9Rot=[]  CS10Pos=[]  CS10Rot=[]  CS11Pos=[]  CS11Rot=[]  CS12Pos=[]  CS12Rot=[]  CS13Pos=[]  CS13Rot=[]  CS14Pos=[]  CS14Rot=[]  CS15Pos=[]  CS15Rot=[]  CS16Pos=[]  CS16Rot=[]  CS17Pos=[]  CS17Rot=[]  CS18Pos=[]  CS18Rot=[]  CS19Pos=[]  CS19Rot=[]  CS20Pos=[]  CS20Rot=[]
      settings: SourceProductName=Simscape Multibody  SourceProductBaseCode=MS
  connections:
  RootPart/RConn1 -- Weld/LConn1
  Weld/RConn1 -- lateral eje y-2/LConn1
  Hombrocopia-1/RConn1 -- Revolute/LConn1
  Revolute/RConn1 -- BASE-1/LConn1
  lateral eje x-2/RConn1 -- Weld1/LConn1
  Weld1/RConn1 -- BASE-1/LConn2
  BASE-1/RConn1 -- Planar/LConn1
  Planar/RConn1 -- mesa-2/LConn1
  lateral eje y-3/RConn1 -- Planar1/LConn1
  Planar1/RConn1 -- BASE-1/LConn3
  lateral eje x-1/RConn1 -- Weld2/LConn1
  Weld2/RConn1 -- BASE-1/LConn4
  Codo-1/RConn1 -- Revolute1/LConn1
  Revolute1/RConn1 -- Antebrazo-1/LConn1
  BrazoCOPIA-1/RConn1 -- Revolute2/LConn1
  Revolute2/RConn1 -- Codo-1/LConn1
  Hombrocopia-1/RConn2 -- Revolute3/LConn1
  Revolute3/RConn1 -- BrazoCOPIA-1/LConn1
  lateral eje x-2/RConn2 -- Prismatic/LConn1
  Prismatic/RConn1 -- mesa-1/LConn1
  lateral eje y-2/RConn1 -- Revolute4/LConn1
  Revolute4/RConn1 -- lateral eje x-2/LConn1
  lateral eje x-1/RConn2 -- Prismatic1/LConn1
  Prismatic1/RConn1 -- lateral eje x-2/LConn2
  mesa-3/RConn1 -- Planar2/LConn1
  Planar2/RConn1 -- mesa-4/LConn1
  lateral eje y-2/RConn2 -- Custom Joint/LConn1
  Custom Joint/RConn1 -- mesa-4/LConn2
  lateral eje y-3/RConn2 -- Cylindrical/LConn1
  Cylindrical/RConn1 -- mesa-4/LConn3
  mesa-2/RConn1 -- Planar3/LConn1
  Planar3/RConn1 -- mesa-3/LConn1
  mesa-1/RConn1 -- Planar4/LConn1
  Planar4/RConn1 -- mesa-2/LConn2
  lateral eje y-3/RConn3 -- Cylindrical1/LConn1
  Cylindrical1/RConn1 -- mesa-2/LConn3
  lateral eje y-2/RConn3 -- Planar5/LConn1
  Planar5/RConn1 -- mesa-3/LConn2
  lateral eje y-3/RConn4 -- Cylindrical2/LConn1
  Cylindrical2/RConn1 -- mesa-3/LConn3
  lateral eje y-3/RConn5 -- Cylindrical3/LConn1
  Cylindrical3/RConn1 -- mesa-1/LConn2
  lateral eje y-2/RConn4 -- Planar6/LConn1
  Planar6/RConn1 -- lateral eje y-3/LConn1
  lateral eje y-2/RConn5 -- Planar7/LConn1
  Planar7/RConn1 -- lateral eje x-1/LConn1
  lateral eje y-3/RConn6 -- Prismatic2/LConn1
  Prismatic2/RConn1 -- lateral eje x-1/LConn2
  RootGround/RConn1 -- Weld3/LConn1
  Weld3/RConn1 -- RootPart/LConn1
  RootGround/LConn1 -- Machine Environment/RConn1
